simulink subsystem "s_sensing"  (R2024b)
settings: Solver=VariableStepAuto  StartTime=0.0  StopTime=10.0  RelTol=1e-3
undefined symbols (not defined in the file): D0, D1, D13, D3, D6, PTA1, PTC16, PTC17, PTC2, PTD1
libraries: frdmk64flib x5
settings Model: Creator=marwa  LastModifiedBy=marwa

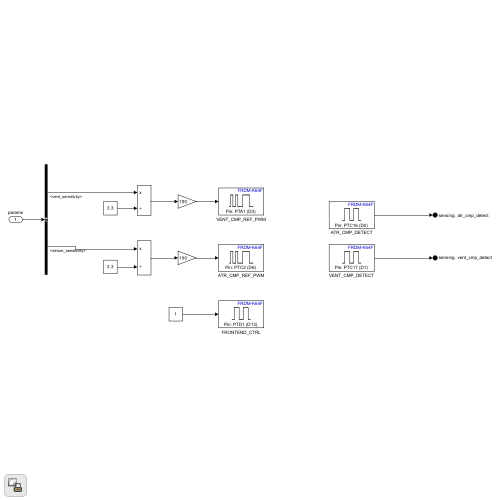
[thumbnail: Simulink's stored preview of the top-level diagram]
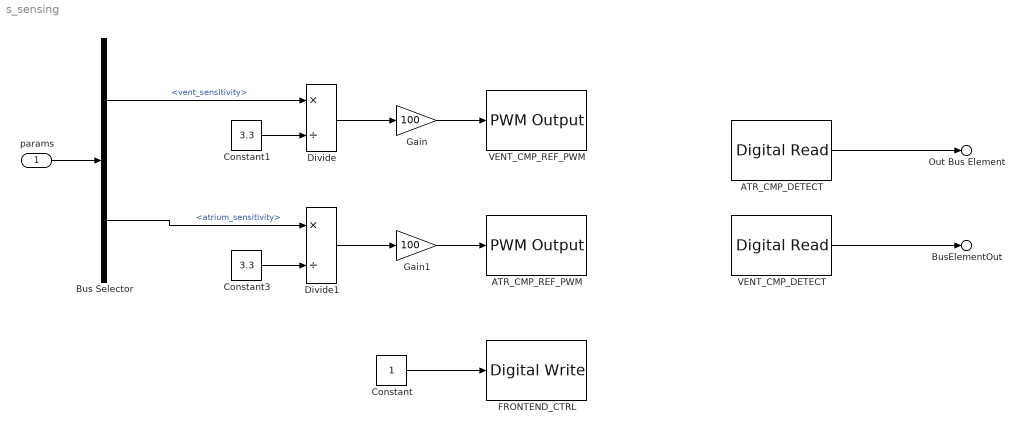
== system s_sensing ==
  params : Inport
  ATR_CMP_DETECT : frdmk64flib/Digital Read  Whichpin=PTC16 (D0)  SampleTime=-1
  ATR_CMP_REF_PWM : frdmk64flib/PWM Output  Whichpin=PTC2 (D6)  InitialFrequency=2000  InitialDutyCycle=0
  Bus Selector : BusSelector  OutputSignals=vent_sensitivity,atrium_sensitivity
  Constant : Constant
  Constant1 : Constant  Value=3.3
  Constant3 : Constant  Value=3.3
  Divide : Product  Inputs=*/
  Divide1 : Product  Inputs=*/
  FRONTEND_CTRL : frdmk64flib/Digital Write  Whichpin=PTD1 (D13)
  Gain : Gain  Gain=100
  Gain1 : Gain  Gain=100
  VENT_CMP_DETECT : frdmk64flib/Digital Read  Whichpin=PTC17 (D1)  SampleTime=-1
  VENT_CMP_REF_PWM : frdmk64flib/PWM Output  Whichpin=PTA1 (D3)  InitialFrequency=2000  InitialDutyCycle=0
  Out Bus Element : Outport  PortName=sensing  Element=atr_cmp_detect
  BusElementOut : Outport  PortName=sensing  Element=vent_cmp_detect
  wires:
  Constant1/1 -> Divide/2
  ATR_CMP_DETECT/1 -> Out Bus Element/1
  Gain/1 -> VENT_CMP_REF_PWM/1
  Constant/1 -> FRONTEND_CTRL/1
  VENT_CMP_DETECT/1 -> BusElementOut/1
  Divide/1 -> Gain/1
  Gain1/1 -> ATR_CMP_REF_PWM/1
  Divide1/1 -> Gain1/1
  Bus Selector/2 -> Divide1/1  "<atrium_sensitivity>"
  Constant3/1 -> Divide1/2
  params/1 -> Bus Selector/1
  Bus Selector/1 -> Divide/1  "<vent_sensitivity>"
